simulink model "bycicle_simulink"  (R2020a)
settings: Solver=ode1  StartTime=0.0  StopTime=Inf  FixedStep=Ts  MaxStep=0.01  RelTol=1e-3
InitFcn:
  | init_bycicle
StopFcn:
  | stop_bycicle
values from neighbouring files (symbols this model uses):
  apertura = 2    [init_bycicle.m]
  centro = [points(1); points(2)]    [init_bycicle.m]
  dir_retta = [1; 0]    [init_bycicle.m]
  K1 = [100	50	10	0	0	0; 	  0		0	0	100	50	10]    [init_bycicle.m]
  K2 = 0.01 * K1    [init_bycicle.m]
  K3 = 0.01 * K1    [init_bycicle.m]
  L = 1    [init_bycicle.m]
  Lsofar = [Lsofar; sum(Lenghts)]    [init_bycicle.m]
  Ltot = sum(Lenghts)    [init_bycicle.m]
  n_p = length(points)    [init_bycicle.m]
  P0 = var_meas * eye(6)    [init_bycicle.m]
  phi_iniziale = 0    [init_bycicle.m]
  s_finale = 1000    [init_bycicle.m]
  theta_P_iniziale = 0    [init_bycicle.m]
  theta_rette = [theta_rette ; theta_rette(n_p-2)+pi]    [init_bycicle.m]
  threshold = 1e-2    (= 0.01)    [init_bycicle.m]
  Ts_filter = 1e-3    (= 0.001)    [init_bycicle.m]
  Ts_meas = 1e-3    (= 0.001)    [init_bycicle.m]
  v_P_dot_iniziale = 0.1    [init_bycicle.m]
  v_P_iniziale = 1    [init_bycicle.m]
  v_r = v_rif    (= 1)    [init_bycicle.m]
  var_meas = (0.001/3)^2    (= 1.11111111111e-07)    [init_bycicle.m]
  x0 = [0; 0; 0; 0]    [FL_biciclo.m]    (also in init_bycicle.m = [x_M_iniziale; y_M_iniziale; phi_iniziale; theta_P_iniziale;)
  x_M_iniziale = points(1)    [init_bycicle.m]
  xp = points(:,1)    [init_bycicle.m]
  y_M_iniziale = points(2)    [init_bycicle.m]
  yp = points(:,2)    [init_bycicle.m]
undefined symbols (not defined in the file or in its folder): indexclot, Lsofarclot
libraries: robotcorelib x2, simulink x1
settings Model: PacingRate=1000  Creator=Andrea_Ferroni  LastModifiedBy=Francesco

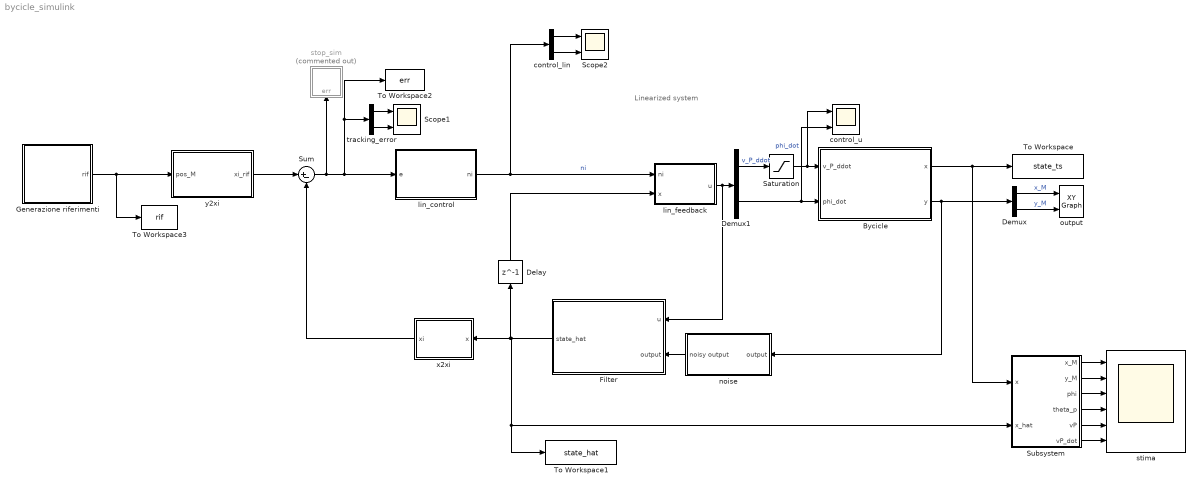
== system bycicle_simulink ==
  note: Linearized system
  Bycicle : Subsystem
      mask Display: image('$imagefile'); % Use "Edit Image" on toolstrip to change.
  Delay : Delay  DelayLength=1  InitialCondition=x0  SampleTime=Ts_filter
  Demux : Demux  Outputs=2
  Demux1 : Demux  Outputs=2
  Filter : Subsystem
  Generazione riferimenti : Subsystem  Variant=on
  Saturation : Saturate  UpperLimit=inf  LowerLimit=-inf
  Scope1 : Scope  NumInputPorts=2
  Scope2 : Scope  NumInputPorts=2
  Subsystem : Subsystem
  Sum : Sum  Inputs=|+-
  To Workspace : ToWorkspace  VariableName=state_ts  SaveFormat=Timeseries  SampleTime=-1
  To Workspace1 : ToWorkspace  VariableName=state_hat  SaveFormat=Timeseries  SampleTime=-1
  To Workspace2 : ToWorkspace  VariableName=err  SaveFormat=Timeseries  SampleTime=-1
  To Workspace3 : ToWorkspace  VariableName=rif  SaveFormat=Timeseries  SampleTime=-1
  control_lin : Demux  Outputs=2
  control_u : Scope  NumInputPorts=2
  lin_control : MATLAB Function  TreatAsAtomicUnit=on
  lin_feedback : MATLAB Function  TreatAsAtomicUnit=on
  noise : Subsystem
  output : simulink/Sinks/XY Graph  xmin=-50  xmax=50  ymin=-50  ymax=50  st=-1
  stima : Scope  NumInputPorts=6
  stop_sim : Subsystem  Commented=on
  tracking_error : Demux  Outputs=2
  x2xi : MATLAB Function  TreatAsAtomicUnit=on
  y2xi : Subsystem
  wires:
  Bycicle/1(x) -> Subsystem/1(x), To Workspace/1
  Bycicle/2(y) -> noise/1(output), Demux/1
  lin_control/1(ni) -> control_lin/1, lin_feedback/1(ni)  "ni"
  Sum/1 -> lin_control/1(e), tracking_error/1, To Workspace2/1, stop_sim/1(err)
  Demux/1 -> output/1  "x_M"
  Demux/2 -> output/2  "y_M"
  tracking_error/1 -> Scope1/1
  tracking_error/2 -> Scope1/2
  lin_feedback/1(u) -> Filter/1(u), Demux1/1
  Demux1/2 -> Bycicle/2(phi_dot), control_u/2  "phi_dot"
  control_lin/2 -> Scope2/2
  control_lin/1 -> Scope2/1
  Generazione riferimenti/1(rif) -> y2xi/1(pos_M), To Workspace3/1
  Saturation/1 -> control_u/1, Bycicle/1(v_P_ddot)
  Demux1/1 -> Saturation/1  "v_P_ddot"
  noise/1(noisy output) -> Filter/2(output)
  y2xi/1(xi_rif) -> Sum/1
  x2xi/1(xi) -> Sum/2
  Filter/1(state_hat) -> Delay/1, x2xi/1(x), To Workspace1/1, Subsystem/2(x_hat)
  Delay/1 -> lin_feedback/2(x)
  Subsystem/1(x_M) -> stima/1
  Subsystem/2(y_M) -> stima/2
  Subsystem/3(phi) -> stima/3
  Subsystem/4(theta_p) -> stima/4
  Subsystem/5(vP) -> stima/5
  Subsystem/6(vP_dot) -> stima/6

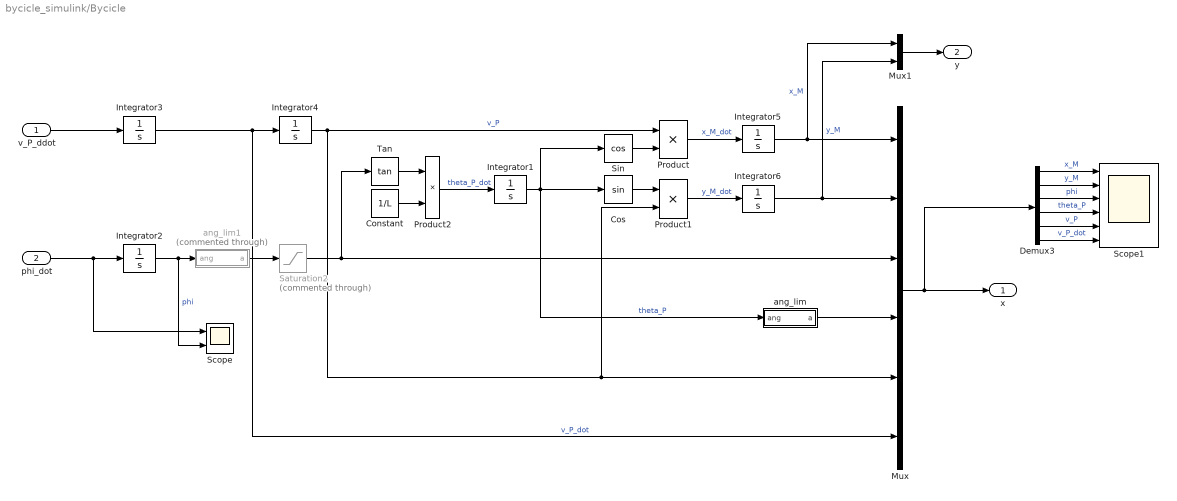
== system bycicle_simulink/Bycicle ==
  v_P_ddot : Inport
  phi_dot : Inport  Port=2
  Constant : Constant  Value=1/L
  Cos : Trigonometry
  Demux3 : Demux  Outputs=6
  Integrator1 : Integrator  InitialCondition=theta_P_iniziale
  Integrator2 : Integrator  InitialCondition=phi_iniziale  LimitOutput=on  UpperSaturationLimit=pi/2  LowerSaturationLimit=-pi/2
  Integrator3 : Integrator  InitialCondition=v_P_dot_iniziale
  Integrator4 : Integrator  InitialCondition=v_P_iniziale
  Integrator5 : Integrator  InitialCondition=x_M_iniziale
  Integrator6 : Integrator  InitialCondition=y_M_iniziale
  Mux : Mux  Inputs=6
  Mux1 : Mux  Inputs=2
  Product : Product
  Product1 : Product
  Product2 : Product
  Saturation2 : Saturate  Commented=through  UpperLimit=pi/2*0.999  LowerLimit=-pi/2*0.999
  Scope : Scope  NumInputPorts=2
  Scope1 : Scope  NumInputPorts=6
  Sin : Trigonometry  Operator=cos
  Tan : Trigonometry  Operator=tan
  ang_lim : MATLAB Function  TreatAsAtomicUnit=on
  ang_lim1 : MATLAB Function  Commented=through  TreatAsAtomicUnit=on
  x : Outport
  y : Outport  Port=2
  wires:
  v_P_ddot/1 -> Integrator3/1
  phi_dot/1 -> Integrator2/1, Scope/1
  Integrator3/1 -> Integrator4/1, Mux/6  "v_P_dot"
  Integrator1/1 -> Sin/1, ang_lim/1(ang), Cos/1  "theta_P"
  Integrator4/1 -> Product1/2, Mux/5, Product/1  "v_P"
  Integrator2/1 -> Scope/2, ang_lim1/1(ang)  "phi"
  Sin/1 -> Product/2
  Cos/1 -> Product1/1
  Product/1 -> Integrator5/1  "x_M_dot"
  Product1/1 -> Integrator6/1  "y_M_dot"
  Tan/1 -> Product2/1
  Constant/1 -> Product2/2
  Product2/1 -> Integrator1/1  "theta_P_dot"
  Mux1/1 -> y/1
  Integrator5/1 -> Mux1/1, Mux/1  "x_M"
  Integrator6/1 -> Mux1/2, Mux/2  "y_M"
  ang_lim/1(a) -> Mux/4
  Saturation2/1 -> Mux/3, Tan/1
  ang_lim1/1(a) -> Saturation2/1
  Demux3/4 -> Scope1/4  "theta_P"
  Demux3/3 -> Scope1/3  "phi"
  Demux3/2 -> Scope1/2  "y_M"
  Demux3/5 -> Scope1/5  "v_P"
  Demux3/1 -> Scope1/1  "x_M"
  Demux3/6 -> Scope1/6  "v_P_dot"
  Mux/1 -> Demux3/1, x/1

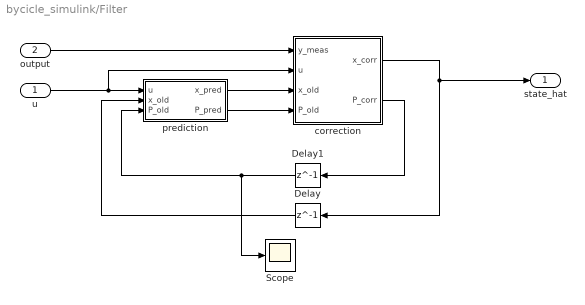
== system bycicle_simulink/Filter ==
  u : Inport
  output : Inport  Port=2
  Delay : Delay  DelayLength=1  InitialCondition=x0  SampleTime=Ts_filter
  Delay1 : Delay  DelayLength=1  InitialCondition=P0  SampleTime=Ts_filter
  Scope : Scope
  correction : MATLAB Function  TreatAsAtomicUnit=on
  prediction : MATLAB Function  TreatAsAtomicUnit=on
  state_hat : Outport
  wires:
  u/1 -> correction/2(u), prediction/1(u)
  correction/1(x_corr) -> state_hat/1, Delay/1
  output/1 -> correction/1(y_meas)
  prediction/1(x_pred) -> correction/3(x_old)
  Delay/1 -> prediction/2(x_old)
  prediction/2(P_pred) -> correction/4(P_old)
  correction/2(P_corr) -> Delay1/1
  Delay1/1 -> Scope/1, prediction/3(P_old)

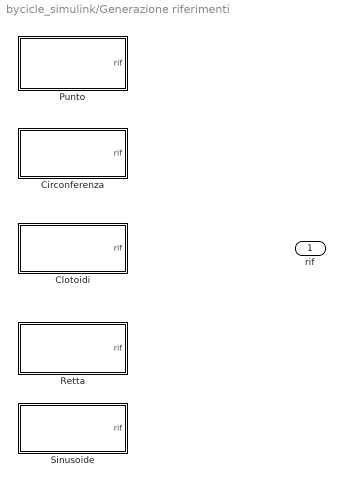
== system bycicle_simulink/Generazione riferimenti ==
  Circonferenza : Subsystem  VariantControl=Circonferenza
  Clotoidi : Subsystem  VariantControl=Clotoidi
  Punto : Subsystem  VariantControl=Punto
  Retta : Subsystem  VariantControl=Retta
  Sinusoide : Subsystem  VariantControl=Sinusoide
  rif : Outport

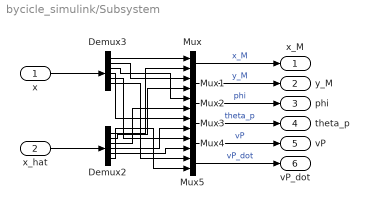
== system bycicle_simulink/Subsystem ==
  x : Inport
  x_hat : Inport  Port=2
  Demux2 : Demux  Outputs=6
  Demux3 : Demux  Outputs=6
  Mux{,1..5} (6 alike) : Mux  Inputs=2
  x_M : Outport
  y_M : Outport  Port=2
  phi : Outport  Port=3
  theta_p : Outport  Port=4
  vP : Outport  Port=5
  vP_dot : Outport  Port=6
  wires:
  Demux2/3 -> Mux2/2
  Demux3/3 -> Mux2/1
  Demux3/4 -> Mux3/1
  Demux3/1 -> Mux/1
  Demux2/2 -> Mux1/2
  Demux2/1 -> Mux/2
  Demux2/6 -> Mux5/2
  Demux3/6 -> Mux5/1
  Demux3/2 -> Mux1/1
  Demux2/4 -> Mux3/2
  Mux5/1 -> vP_dot/1  "vP_dot"
  Demux3/5 -> Mux4/1
  Demux2/5 -> Mux4/2
  Mux1/1 -> y_M/1  "y_M"
  x/1 -> Demux3/1
  Mux/1 -> x_M/1  "x_M"
  x_hat/1 -> Demux2/1
  Mux4/1 -> vP/1  "vP"
  Mux2/1 -> phi/1  "phi"
  Mux3/1 -> theta_p/1  "theta_p"

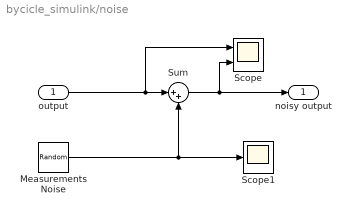
== system bycicle_simulink/noise ==
  output : Inport
  Measurements Noise : RandomNumber  Variance=var_meas  Seed=[10, 13]  SampleTime=Ts_meas
  Scope : Scope  NumInputPorts=2
  Scope1 : Scope
  Sum : Sum  Inputs=|++
  noisy output : Outport
  wires:
  output/1 -> Scope/1, Sum/1
  Sum/1 -> Scope/2, noisy output/1
  Measurements Noise/1 -> Scope1/1, Sum/2

== system bycicle_simulink/stop_sim ==
  err : Inport
  Delay : Delay  DelayLength=1
  MATLAB Function1 : MATLAB Function  TreatAsAtomicUnit=on
  Stop Simulation : Stop
  wires:
  MATLAB Function1/2(n) -> Delay/1
  MATLAB Function1/1(flag) -> Stop Simulation/1
  err/1 -> MATLAB Function1/1(err)
  Delay/1 -> MATLAB Function1/2(n_old)

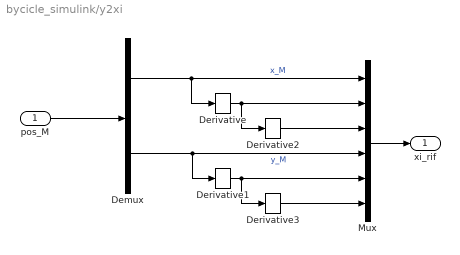
== system bycicle_simulink/y2xi ==
  pos_M : Inport
  Demux : Demux  Outputs=2
  Derivative{,1..3} (4 alike) : Derivative  CoefficientInTFapproximation=1e10
  Mux : Mux  Inputs=6
  xi_rif : Outport
  wires:
  pos_M/1 -> Demux/1
  Mux/1 -> xi_rif/1
  Demux/1 -> Derivative/1, Mux/1  "x_M"
  Demux/2 -> Derivative1/1, Mux/4  "y_M"
  Derivative1/1 -> Derivative3/1, Mux/5
  Derivative/1 -> Mux/2, Derivative2/1
  Derivative2/1 -> Mux/3
  Derivative3/1 -> Mux/6

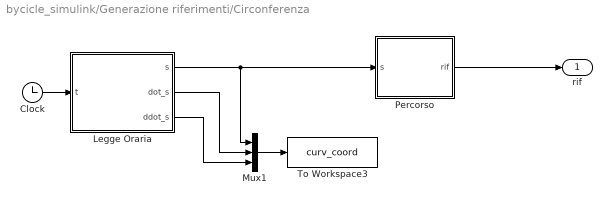
== system bycicle_simulink/Generazione riferimenti/Circonferenza ==
  Clock : Clock
  Legge Oraria : MATLAB Function  TreatAsAtomicUnit=on
  Mux1 : Mux  Inputs=3
  Percorso : MATLAB Function  TreatAsAtomicUnit=on
  To Workspace3 : ToWorkspace  VariableName=curv_coord  SaveFormat=Timeseries  SampleTime=-1
  rif : Outport
  wires:
  Legge Oraria/2(dot_s) -> Mux1/2
  Clock/1 -> Legge Oraria/1(t)
  Mux1/1 -> To Workspace3/1
  Legge Oraria/3(ddot_s) -> Mux1/3
  Legge Oraria/1(s) -> Percorso/1(s), Mux1/1
  Percorso/1(rif) -> rif/1

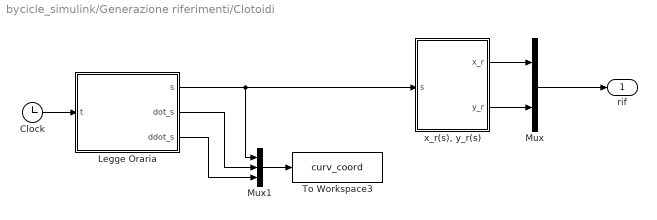
== system bycicle_simulink/Generazione riferimenti/Clotoidi ==
  Clock : Clock
  Legge Oraria : MATLAB Function  TreatAsAtomicUnit=on
  Mux : Mux  Inputs=2
  Mux1 : Mux  Inputs=3
  To Workspace3 : ToWorkspace  VariableName=curv_coord  SaveFormat=Timeseries  SampleTime=-1
  "x_r(s), y_r(s)" : MATLAB Function  TreatAsAtomicUnit=on
  rif : Outport
  wires:
  Legge Oraria/1(s) -> Mux1/1, "x_r(s), y_r(s)"/1(s)
  Legge Oraria/2(dot_s) -> Mux1/2
  Clock/1 -> Legge Oraria/1(t)
  Legge Oraria/3(ddot_s) -> Mux1/3
  Mux1/1 -> To Workspace3/1
  "x_r(s), y_r(s)"/2(y_r) -> Mux/2
  "x_r(s), y_r(s)"/1(x_r) -> Mux/1
  Mux/1 -> rif/1

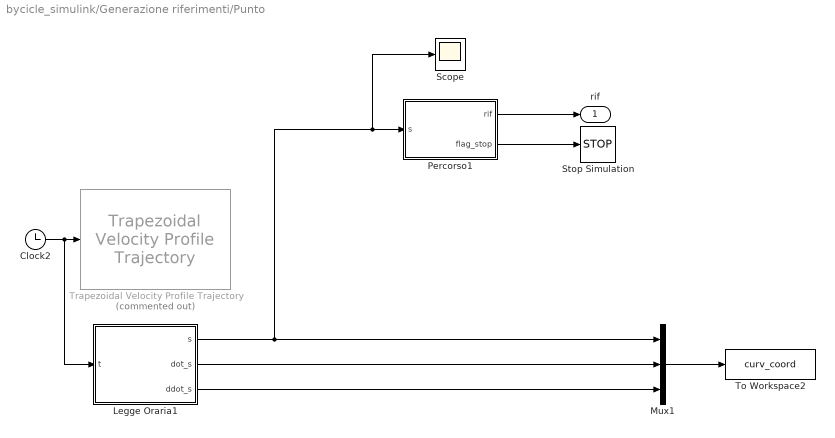
== system bycicle_simulink/Generazione riferimenti/Punto ==
  Clock2 : Clock
  Legge Oraria1 : MATLAB Function  TreatAsAtomicUnit=on
  Mux1 : Mux  Inputs=3
  Percorso1 : MATLAB Function  TreatAsAtomicUnit=on
  Scope : Scope
  Stop Simulation : Stop
  To Workspace2 : ToWorkspace  VariableName=curv_coord  SaveFormat=Timeseries  SampleTime=-1
  Trapezoidal Velocity Profile Trajectory : robotcorelib/Trapezoidal Velocity Profile Trajectory  Commented=on  WaypointSource=Internal  Waypoints="[ 0,  s_finale]"  NumParams=1  Parameter1=Peak Velocity  Parameter2=End Time  ParameterSource=Internal  PeakVelocity=v_rif  Acceleration=a_rif  EndTime=[ 1; 1 ]  AccelTime=[ 1; 2 ]  SimulateUsing=Interpreted execution
      settings: SourceProductBaseCode=NV,RO,RR
  rif : Outport
  wires:
  Clock2/1 -> Legge Oraria1/1(t), Trapezoidal Velocity Profile Trajectory/1
  Percorso1/1(rif) -> rif/1
  Mux1/1 -> To Workspace2/1
  Legge Oraria1/1(s) -> Mux1/1, Scope/1, Percorso1/1(s)
  Legge Oraria1/2(dot_s) -> Mux1/2
  Legge Oraria1/3(ddot_s) -> Mux1/3
  Percorso1/2(flag_stop) -> Stop Simulation/1

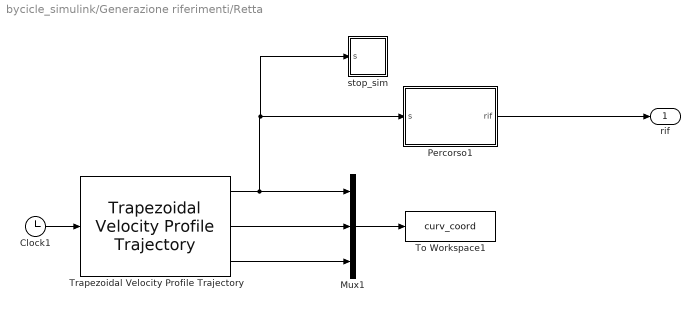
== system bycicle_simulink/Generazione riferimenti/Retta ==
  Clock1 : Clock
  Mux1 : Mux  Inputs=3
  Percorso1 : MATLAB Function  TreatAsAtomicUnit=on
  To Workspace1 : ToWorkspace  VariableName=curv_coord  SaveFormat=Timeseries  SampleTime=-1
  Trapezoidal Velocity Profile Trajectory : robotcorelib/Trapezoidal Velocity Profile Trajectory  WaypointSource=Internal  Waypoints="[ 0,  s_finale]"  NumParams=2  Parameter1=Peak Velocity  Parameter2=Acceleration  ParameterSource=Internal  PeakVelocity=v_rif  Acceleration=a_rif  EndTime=[ 1; 1 ]  AccelTime=[ 1; 2 ]  SimulateUsing=Interpreted execution
      settings: SourceProductBaseCode=NV,RO,RR
  stop_sim : Subsystem
  rif : Outport
  wires:
  Trapezoidal Velocity Profile Trajectory/1 -> stop_sim/1(s), Percorso1/1(s), Mux1/1
  Mux1/1 -> To Workspace1/1
  Percorso1/1(rif) -> rif/1
  Clock1/1 -> Trapezoidal Velocity Profile Trajectory/1
  Trapezoidal Velocity Profile Trajectory/2 -> Mux1/2
  Trapezoidal Velocity Profile Trajectory/3 -> Mux1/3

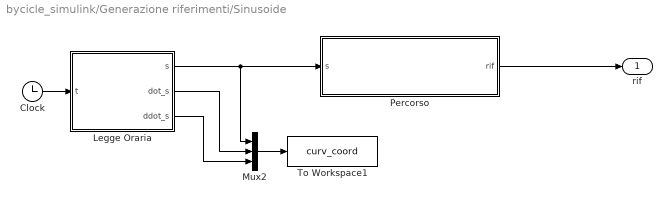
== system bycicle_simulink/Generazione riferimenti/Sinusoide ==
  Clock : Clock
  Legge Oraria : MATLAB Function  TreatAsAtomicUnit=on
  Mux2 : Mux  Inputs=3
  Percorso : MATLAB Function  TreatAsAtomicUnit=on
  To Workspace1 : ToWorkspace  VariableName=curv_coord  SaveFormat=Timeseries  SampleTime=-1
  rif : Outport
  wires:
  Legge Oraria/2(dot_s) -> Mux2/2
  Clock/1 -> Legge Oraria/1(t)
  Mux2/1 -> To Workspace1/1
  Legge Oraria/3(ddot_s) -> Mux2/3
  Legge Oraria/1(s) -> Mux2/1, Percorso/1(s)
  Percorso/1(rif) -> rif/1

== system bycicle_simulink/Generazione riferimenti/Retta/stop_sim ==
  s : Inport
  Delay : Delay  DelayLength=1
  MATLAB Function1 : MATLAB Function  TreatAsAtomicUnit=on
  Stop Simulation : Stop
  wires:
  MATLAB Function1/2(n) -> Delay/1
  MATLAB Function1/1(flag) -> Stop Simulation/1
  s/1 -> MATLAB Function1/1(s)
  Delay/1 -> MATLAB Function1/2(n_old)

== matlab function bycicle_simulink/Bycicle/ang_lim1 ==
  data: ang input; a output
function a = ang_lim(ang)

	c = cos(ang);
	s = sin(ang);
	a = atan2(s, c);

end

== matlab function bycicle_simulink/Generazione riferimenti/Circonferenza/Legge Oraria ==
  data: t input; s output; v_rif parameter; dot_s output; ddot_s output
function [s, dot_s, ddot_s]  = legge_oraria(t, v_rif)
%#codegen PEPO

s = v_rif*t;
dot_s = v_rif;
ddot_s = 0.0;


end

== matlab function bycicle_simulink/Generazione riferimenti/Circonferenza/Percorso ==
  data: s input; rif output; centro parameter; v_r parameter
function rif = percorso(s, centro, v_r)

r = 10*v_r;  % 1
theta_circ = s/r;

if theta_circ >=  3*2*pi % dopotre giri ti fermi
	theta_circ = 3*2*pi;
end

rif = centro + r*[cos(theta_circ);sin(theta_circ)];		% circonferenza

end

== matlab function bycicle_simulink/Filter/prediction ==
  data: u input; x_old input; x_pred output; P_old input; P_pred output; L parameter; Ts_filter parameter
function [x_pred, P_pred] = pred(u, x_old, P_old, L, Ts_filter)

[x_pred, P_pred] = ukf_predict(x_old, P_old, u, L, Ts_filter);

end

%%%%%%%%%%%%%%%%%%%%%%%%%

function [x_new, P_new] = ukf_predict(x_old, P_old, u, L, Ts_filter)
 % ukf_predict generates 2n+1 sigma points, it propagates them using
 % state_update and outputs the mean and the covariance of the new sigma 
 % points distribution. 
 %
 % Input		
 % x_old		old state vector nx1
 % P_old		old state covariance matrix nxn
 % u			input vector px1
 %
 % Output
 % x_new		new state vector nx1
 % P_new		new state covariance matrix nxn

 %generation of sigma points and weights
[sp, wm, wc] = sigmapoint_gen(x_old, P_old);

%propagation using state update function
[x_new, P] = sigmapoint_propagate(sp, wm, wc, u, L, Ts_filter);

% forced simmetry
P_new = (P + P')/2;

end

%--------------------------------------------------------------------------
%--------------------------------------------------------------------------
function [sp, wm, wc] = sigmapoint_gen(x_old, P_old)
% function that generates sigma points and weights

	n		= size(x_old,1);	% state dimension in which sigma points are generated
	nsp		= 2*n+1;			% number of sigma points
	P       = P_old;			% covariance matrix
	
	% parameters for simmetric distribution
	alpha	= 1;
	beta	= 2;
	k		= 0;
    
	lambda = alpha^2 * (n + k) -n;
	
	% generation of first order weights (weights mean)
	wm = 1/(2*(n + lambda)) * ones(nsp, 1);
    wm(1) = lambda/(n + lambda);
	
	% generation of second order weights (weights covariance)
	wc = 1/(2*(n + lambda)) * ones(nsp, 1);
	wc(1) = lambda/(n + lambda) + (1 - alpha^2 + beta);
	
	% generation sigma points sp
	dist	= zeros(n,n);
	sp		= zeros(n, nsp);
	
	% calculation of dist = sqrt((n+lambda)*P)
	[U, SIGMA, ~] = svd((n+lambda)* P);
	dist = U * sqrt(SIGMA);

	for i=1:nsp
		if i == 1
			sp(:,i) = x_old;
		elseif i <= 1+n
			sp(:,i) = x_old + dist(:,i-1);
		elseif i > 1+n && i<=nsp
			sp(:,i) = x_old - dist(:,i-1-n);
		end
	end

end

%--------------------------------------------------------------------------
%--------------------------------------------------------------------------
function [x_new, P_new] = sigmapoint_propagate(sp, wm, wc, u, L, Ts_filter)
% this function, using state_update, propagates the sp distribution
	
	n = size(sp(:,1),1);	% state dimension
	nsp = n*2 + 1;			% number of sigma points
	
	% init of the new sp distribution
	sp_new = zeros(n, nsp);	
	
	% propagation
	for j = 1:nsp
		 sp_new(:,j) = state_update(sp(:,j), u, L, Ts_filter);
	end
	
	%%ANGLE in state

	% note: to correctly compute mean and covariance of angular entity is 
	% better to obtain first the mean of cosin and sin and
	% then obtain the mean angle using atan2

	mean_c = zeros(n, 1);	% cosin mean
	mean_s = zeros(n, 1);	% sin mean
	for j = 1:nsp
		c = cos(sp_new(:,j));
		s = sin(sp_new(:,j));

		mean_c = mean_c + wm(j)*c;
		mean_s = mean_s + wm(j)*s;
	end

	x_new_a = atan2(mean_s, mean_c); % atan2 of mean

	% cov
	cc = zeros(n,n);		% cosin covariance
	cs = zeros(n,n);		% sin covariance
	for j = 1:nsp
		c = cos(sp_new(:,j) - x_new_a);
		s = sin(sp_new(:,j) - x_new_a);

		cc = cc + wc(j)*(c*c');
		cs = cs + wc(j)*(s*s');
	end
	P_new_a = atan2(cs,cc);	% atan2 of covariance


	% no angle in state
	%mean
	mean = zeros(n, 1);
	for j = 1:nsp
		mean = mean + wm(j)*sp_new(:,j);
	end
	x_new_na = mean;
	% covar
	covar = zeros(n,n);
	for j = 1:nsp
		covar = covar + wc(j)*((sp_new(:,j) - x_new_na)*(sp_new(:,j) - x_new_na)');
	end
	
	P_new_na = covar;

	x_new = [x_new_na(1:2, 1);		x_new_a(3:4, 1);	x_new_na(5:6, 1)];
	%P_new = [P_new_na(1:2, 1:2);	P_new_a(3:4, 3:4);	P_new_na(5:6, 5:6)];
	P_new = P_new_na;
	P_new(3,:) = P_new_a(3,:);
	P_new(4,:) = P_new_a(4,:);
	P_new(:,3) = P_new_a(:,3);
	P_new(:,4) = P_new_a(:,4);
end

%--------------------------------------------------------------------------
%--------------------------------------------------------------------------
function x_new = state_update(x_old, u, L, Ts_filter)
% state_update Local function that calculates how the state updates.

	
	x_M		= x_old(1);
	y_M		= x_old(2);
	phi		= x_old(3);
	theta_P = x_old(4);
	v_P		= x_old(5);
	v_P_dot = x_old(6);

	f_x_old = [ v_P*cos(theta_P)	;...
				v_P*sin(theta_P)	;...
                0					;...
				(v_P*tan(phi))/L	;...
				v_P_dot				;...
                0					];					
				
	g = [	0     0	;...
			0     0 ;...
			0     1 ;...
			0     0 ;...
			0     0 ;...
			1     0	];
     
	
    x_new = x_old + (f_x_old + g*u) * Ts_filter ;
end
 
 
%%

== matlab function bycicle_simulink/Filter/correction ==
  data: y_meas input; u input; x_old input; x_corr output; P_old input; P_corr output; R parameter
function [x_corr, P_corr] = corr(y_meas, u, x_old, P_old, R)

[y_virt, S_virt, C] = ukf_virtmeas(x_old, P_old, u);

e = y_meas - y_virt;
S = S_virt + R;

[x_corr, P_corr]= ukf_correct(x_old, P_old, e, S, C);

end

%%%%%%%%%%%%%%%%%%%%%%%%%
function [x_new, P_new]= ukf_correct(x_old, P_old, e, S, C)
	% filter correction, using Kalman theory
	
	K = C*(inv(S)); 
    P_delta = - K*S*K';
	
    x_new = x_old + K*e;
    P = P_old + P_delta;    
	
	P_new = (P+P')/2; % forced simmetry
end

%%%%%%%%%%%%%%%%%%%%%%%%%
function [y_virt, S_virt, C] = ukf_virtmeas(x, P, u)
 % ukf_virtmeas generates 2n+1 sigma points, it propagates them using
 % state2meas and outputs the mean and the covariance of the new sigma 
 % points distribution and the crosscorelation between state and virtual 
 % measurements. 
 %
 % Input		
 % x			state vector nx1
 % P			state covariance matrix nxn
 % u			input vector px1
 %
 % Output
 % y_virt		virtual measurements vector mx1
 % S_virt		virtual measurements covariance matrix mxm
 % C			state-measurements crosscorelation matrix nxm
 
% generation of sigmapoints and their weights
[sp, wm, wc] = sigmapoint_gen(x, P);

% propagation of state vector using state2meas
[~, y_virt, esse, C] = spstate2meas(sp, x, wm, wc, u);

% forced simmetry							
S_virt = (esse + esse')/2;

end

%--------------------------------------------------------------------------
%--------------------------------------------------------------------------
function [sp, wm, wc] = sigmapoint_gen(x, P)
% function that generates sigma points and weights

	n		= size(x,1);		% state dimension in which sigma points are generated
	nsp		= 2*n+1;			% number of sigma points
	P       = P;				% covariance matrix
	
	% parameters for simmetric distribution
	alpha	= 1;
	beta	= 2;
	k		= 0;
    
	lambda = alpha^2 * (n + k) -n;
	
	% generation of first order weights (weights mean)
	wm = 1/(2*(n + lambda)) * ones(nsp, 1);
    wm(1) = lambda/(n + lambda);
	
	% generation of second order weights (weights covariance)
	wc = 1/(2*(n + lambda)) * ones(nsp, 1);
	wc(1) = lambda/(n + lambda) + (1 - alpha^2 + beta);
	
	% generation sigma points sp
	dist	= zeros(n,n);
	sp		= zeros(n, nsp);
	
	% computation of dist = sqrt((n+lambda)*P)
	[U, SIGMA, ~] = svd((n+lambda)* P);
	dist = U * sqrt(SIGMA);

	for i=1:nsp
		if i == 1
			sp(:,i) = x;
		elseif i <= 1+n
			sp(:,i) = x + dist(:,i-1);
		elseif i > 1+n && i<=nsp
			sp(:,i) = x - dist(:,i-1-n);
		end
	end


end

%--------------------------------------------------------------------------
%--------------------------------------------------------------------------
function [sp_meas_new, y_virt, S_new, C] = spstate2meas(sp, x, wm, wc, u)
% this function propagates sigmapoint using state2meas and then computes
% mean, covariance matrix and crosscorelation matrix
	
	n  = size(x,1);		% state dimension
	nsp = 2*n + 1;		% number of sigma points
	
	% init sigma points propagated
	n_meas = size(state2meas(x, u),1);
	sp_meas_new = zeros(n_meas, nsp);
	
	% propagation through meas function
	for j = 1:nsp
		sp_meas_new(:,j) = state2meas(sp(:,j),u);
	end
	
	% virt meas mean
	y_virt = zeros(n_meas, 1);
	for j = 1:nsp
		y_virt = y_virt + wm(j)*sp_meas_new(:,j);
	end

	% virt meas matrix covariance
	S_new = zeros(n_meas, n_meas);  
	for j = 1:nsp
		 S_new = S_new + wc(j)*(sp_meas_new(:,j) - y_virt)*(sp_meas_new(:,j) - y_virt)';
	end
	
	% crosscov state - meas virt
	C_a		= zeros(n, n_meas);
	% angles in the state
	for j = 1:nsp
		% angular difference obtained from cosin and sin of difference
		% between angles
		ang = (sp(:,j)-x);				% angle diff
		a = atan2(sin(ang),cos(ang));	% atan2 of angle diff

		C_a = C_a + wc(j)*( a * (sp_meas_new(:,j)- y_virt(:,1))');
	end
	
	% no angle in the state
	C_na	= zeros(n, n_meas);
	for j = 1:nsp
		diff = (sp(:,j)-x);
		C_na = C_na + wc(j)*( diff * (sp_meas_new(:,j)- y_virt(:,1))');
	end
	
	C	= C_na;
	C(3:4,:) = C_a(3:4,:);
end

%%%%%%%%%%%%%%%%%%%%%%%%%
function y = state2meas(x, u)
% state2meas function that calculates outputs given state.
	
    y = [x(1); x(2)];
end

== matlab function bycicle_simulink/Generazione riferimenti/Clotoidi/x_r(s), y_r(s) ==
  data: s input; x_r output size=1; y_r output size=1; indexclot parameter; theta_rette parameter; yp parameter; xp parameter; Lsofar parameter; n_p parameter; Lsofarclot parameter; Ltot parameter
function [x_r,y_r] = percorso(s, indexclot, theta_rette, yp, xp, ...
										Lsofar, n_p, Lsofarclot, Ltot)
									
coder.extrinsic('pointsOnClothoid')
% fine percorso
if s >= Ltot
	s = Ltot; % cosi` da plottare l'ultimo punto
end

ntratto=0;
	XYS = [0; 0]; %definito prima

	%Parte per capire in che tratto sono
	if s < Lsofar(1)
		ntratto=1;
	else
		for ii=2:(n_p-1)
			if s>=Lsofar(ii-1) && s<=Lsofar(ii)
				ntratto=ii;
			end
		end
	end	

		%calcolo delle coordinate x e y riferite a s e a ntratto
	if mod(ntratto,2)==1            %tratti dispari - rette
		if ntratto==1
			XYS=[xp(ntratto)+cos(theta_rette(ntratto))*(s); ...
				yp(ntratto)+sin(theta_rette(ntratto))*(s)];
		else
			srel=s-Lsofar(ntratto-1);
			XYS=[	xp(ntratto)	+ cos(theta_rette(ntratto))	* srel; ...
					yp(ntratto)	+ sin(theta_rette(ntratto))	* srel];
		end 

	elseif mod(ntratto,2)==0	%tratti pari - clotoidi
		srel=s-Lsofar(ntratto-1);

		if srel<=Lsofarclot(ntratto/2).Lclot(1)
			XYS = double(pointsOnClothoid( indexclot(ntratto/2).clot.S0, srel ));

		elseif srel>Lsofarclot(ntratto/2).Lclot(1) & srel<=Lsofarclot(ntratto/2).Lclot(2)
			XYS = double(pointsOnClothoid( indexclot(ntratto/2).clot.SM, srel- indexclot(ntratto/2).clot.S0.L ));

		elseif srel>Lsofarclot(ntratto/2).Lclot(2)
			XYS = double(pointsOnClothoid( indexclot(ntratto/2).clot.S1, srel- indexclot(ntratto/2).clot.S0.L - indexclot(ntratto/2).clot.SM.L ));
		end

		%XYS = double(pointsOnClothoid( indexclot(ntratto/2).clot, s-Lsofar(ntratto-1) ));
	end

	x_r = XYS(1);
	y_r = XYS(2);
%--------------------------------------------------
% end function
end

== matlab function bycicle_simulink/Generazione riferimenti/Sinusoide/Legge Oraria ==
  data: t input; s output; v_rif parameter; dot_s output; ddot_s output
function [s, dot_s, ddot_s]  = legge_oraria(t, v_rif)
%#codegen PEPO

s = v_rif*t;
dot_s = v_rif;
ddot_s = 0.0;


end

== matlab function bycicle_simulink/Generazione riferimenti/Sinusoide/Percorso ==
  data: s input; rif output; dir_retta parameter; apertura parameter
function rif  = retta(s, dir_retta, apertura)

r = 5;
theta_circ = s/r/apertura;

% if theta_circ >=  3*2*pi % dopotre giri ti fermi
% 	theta_circ = 3*2*pi;
% end

rif = dir_retta * s + r*[0; sin(theta_circ)];	% circonferenza

end

== matlab function bycicle_simulink/Generazione riferimenti/Punto/Legge Oraria1 ==
  data: t input; s output; v_rif parameter; dot_s output; ddot_s output
function [s, dot_s, ddot_s]  = legge_oraria(t, v_rif)
%#codegen PEPO

s = v_rif*t;
dot_s = v_rif;
ddot_s = 0.0;


end

== matlab function bycicle_simulink/x2xi ==
  data: x input; xi output; L parameter
function xi = x2xi(x, L)

x_M		= x(1);
y_M		= x(2);
phi		= x(3);
theta_P = x(4);
v_P		= x(5);
v_P_dot = x(6);


xi = [												x_M;...
                                       v_P*cos(theta_P);...
 v_P_dot*cos(theta_P) - (v_P^2*tan(phi)*sin(theta_P))/L;...
                                                    y_M;...
                                       v_P*sin(theta_P);...
 (cos(theta_P)*tan(phi)*v_P^2)/L + v_P_dot*sin(theta_P)];
	


end

== matlab function bycicle_simulink/Generazione riferimenti/Punto/Percorso1 ==
  data: s input; rif output; dir_retta parameter; x_M_iniziale parameter; y_M_iniziale parameter; s_finale parameter; flag_stop output
function [rif, flag_stop] = retta(s, dir_retta, x_M_iniziale, y_M_iniziale, s_finale)

if s >= s_finale
	s = s_finale;
	flag_stop = 1;
else
	flag_stop = 0;
end

rif = [x_M_iniziale; y_M_iniziale] + s * dir_retta;




end

== matlab function bycicle_simulink/lin_control ==
  data: e input; ni output; K1 parameter; K2 parameter; K3 parameter
function ni = lin_control(e, K1, K2, K3)


% edot = e_dot(1:6,1);
% eddot = e_dot(7:12,1);
% ni = K1*e + K2*edot + K3*eddot;

ni = K1*e;

end

== matlab function bycicle_simulink/lin_feedback ==
  data: ni input; x input; u output; L parameter
function u = Linearized(ni, x,L)
E_inv	= inv_E(x,L);
G		= Gamma(x,L);
u		=  -E_inv*G + E_inv*ni;
end

% gamma
function Gm = Gamma(x,L)
phi = x(3);
theta_P = x(4);
v_P = x(5);
v_P_dot = x(6);

Gm =  [- (v_P*tan(phi)*((cos(theta_P)*tan(phi)*v_P^2)/L + v_P_dot*sin(theta_P)))/L - (2*v_P*v_P_dot*tan(phi)*sin(theta_P))/L;...
		 (v_P*tan(phi)*(v_P_dot*cos(theta_P) - (v_P^2*tan(phi)*sin(theta_P))/L))/L + (2*v_P*v_P_dot*cos(theta_P)*tan(phi))/L];
end
% 
function E_in = inv_E(x,L)
phi		= x(3);
theta_P = x(4);
v_P		= x(5);

E =[cos(theta_P), -(v_P^2*sin(theta_P)*(tan(phi)^2 + 1))/L;...
	sin(theta_P),  (v_P^2*cos(theta_P)*(tan(phi)^2 + 1))/L];


% if rcond(E) < 1e-5
% 	ciao = 1;
% end

E_in = inv(E);


end

== matlab function bycicle_simulink/Generazione riferimenti/Retta/Percorso1 ==
  data: s input; rif output; dir_retta parameter
function rif  = retta(s, dir_retta)

rif = s * dir_retta;

end

== matlab function bycicle_simulink/Bycicle/ang_lim ==
  data: ang input; a output
function a = ang_lim(ang)

	c = cos(ang);
	s = sin(ang);
	a = atan2(s, c);

end

== matlab function bycicle_simulink/stop_sim/MATLAB Function1 ==
  data: flag output; err input; n output; n_old input; threshold parameter
function [flag, n] = stop_function(err, n_old, threshold)
	flag = 0;
	n = n_old;
	if norm(err, 2) < threshold
		n=n+1;
	else
		n=0;
	end
	
	if n > 500
		flag = 1;
		n = 0;
	end
end

== matlab function bycicle_simulink/Generazione riferimenti/Retta/stop_sim/MATLAB Function1 ==
  data: flag output; s input; n output; n_old input; threshold parameter; s_finale parameter
function [flag, n] = stop_function(s, n_old, threshold, s_finale)
	flag = 0;
	n = n_old;
	if norm(s-s_finale, 2) < threshold
		n=n+1;
	else
		n=0;
	end
	
	if n > 100
		flag = 1;
		n = 0;
	end
end

== matlab function bycicle_simulink/Generazione riferimenti/Clotoidi/Legge Oraria ==
  data: t input; s output; v_rif parameter; dot_s output; ddot_s output
function [s, dot_s, ddot_s]  = legge_oraria(t, v_rif)
%#codegen PEPO

s = v_rif*t;
dot_s = v_rif;
ddot_s = 0.0;


end
